simulink model "A12_3_v2018_blagodaram_Ana"  (R2018a)
settings: Solver=ode45  StartTime=0.0  StopTime=300  RelTol=1e-3  EnableMultiTasking=on
libraries: simulink x2
settings Model: Creator=Gorjan  LastModifiedBy=Ana Sofronievska
settings DataIOCC: LimitDataPoints=on  SaveFormat=Array
settings OptimizationCC: LifeSpan=inf
settings DebuggingCC: UnderspecifiedInitializationDetection=Classic  MergeDetectMultiDrivingBlocksExec=none  SolverPrmCheckMsg=warning  StateNameClashWarn=warning  SFUnexpectedBacktrackingDiag=warning  SFNoUnconditionalDefaultTransitionDiag=warning  SFExecutionAtInitializationDiag=none
settings HardwareCC: ProdBitPerPointer=32  ProdBitPerSizeT=32  ProdBitPerPtrDiffT=32  ProdLargestAtomicFloat=None  ProdIntDivRoundTo=Undefined  ProdEndianess=Unspecified  ProdWordSize=32  ProdHWDeviceType=32-bit Generic
settings ModelReferenceCC: PropagateSignalLabelsOutOfModel=off
settings CodeAppCC: StateflowObjectComments=on
settings GRTTargetCC: TargetLangStandard=C89/C90 (ANSI)
settings ConfigComp: CovMetricSettings=dw  CovSaveCumulativeToWorkspaceVar=on  CovSaveSingleToWorkspaceVar=on  CovExternalEMLEnable=off

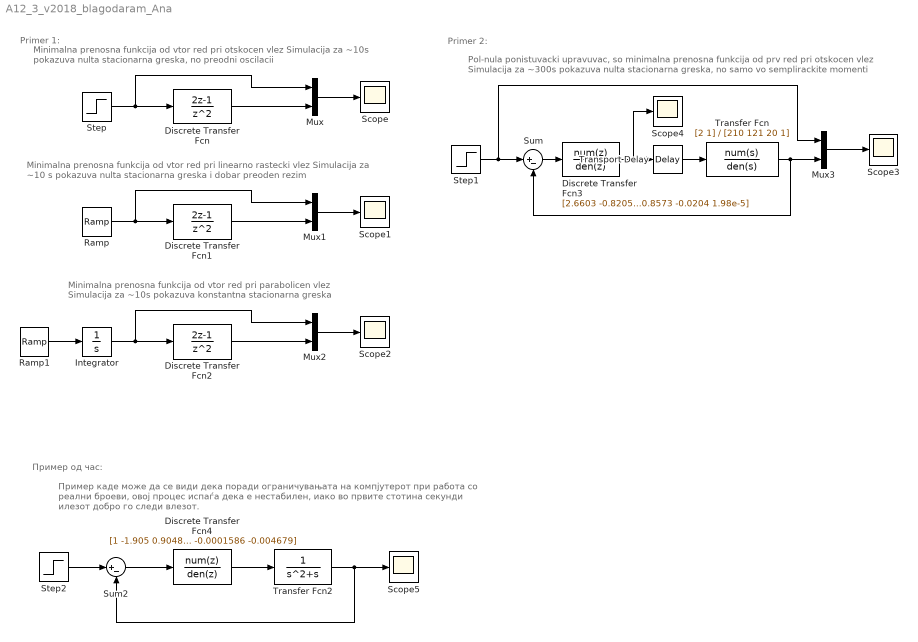
== system A12_3_v2018_blagodaram_Ana ==
  note: Primer 2:
  note: Primer 1:
  note: Minimalna prenosna funkcija od vtor red pri otskocen vlez
      | Simulacija za ~10s pokazuva nulta stacionarna greska, no preodni oscilacii
  note: Minimalna prenosna funkcija od vtor red pri linearno rastecki vlez
      | Simulacija za ~10 s pokazuva nulta stacionarna greska i dobar preoden rezim
  note: Minimalna prenosna funkcija od vtor red pri parabolicen vlez
      | Simulacija za ~10s pokazuva konstantna stacionarna greska
  note: Pol-nula ponistuvacki upravuvac, so minimalna prenosna funkcija od prv red pri otskocen vlez
      | Simulacija za ~300s pokazuva nulta stacionarna greska, no samo vo semplirackite momenti
  note: Пример од час:
  note: Пример каде може да се види дека поради ограничувањата на компјутерот при работа со реални броеви, овој процес испаѓа дека е нестабилен, иако во првите стотина секунди илезот добро го следи влезот.
  Discrete Transfer Fcn : DiscreteTransferFcn  Numerator=[2 -1]  Denominator=[1 0 0]  SampleTime=1
  Discrete Transfer Fcn1 : DiscreteTransferFcn  Numerator=[2 -1]  Denominator=[1 0 0]  SampleTime=1
  Discrete Transfer Fcn2 : DiscreteTransferFcn  Numerator=[2 -1]  Denominator=[1 0 0]  SampleTime=1
  Discrete Transfer Fcn3 : DiscreteTransferFcn  Numerator=[2.6603 -0.8205 0.0585 -2.64e-4 0]  Denominator=[1 -0.1223 -0.8573 -0.0204 1.98e-5]  SampleTime=16
  Discrete Transfer Fcn4 : DiscreteTransferFcn  Numerator=[1 -1.905 0.9048]  Denominator=[0.004837 -0.0001586 -0.004679]  SampleTime=0.1
  Integrator : Integrator
  Mux{,1..3} (4 alike) : Mux  Inputs=2
  Ramp : simulink/Sources/Ramp  slope=1  start=0  InitialOutput=0
  Ramp1 : simulink/Sources/Ramp  slope=1  start=0  InitialOutput=0
  Scope{,1..5} (6 alike) : Scope
  Step : Step  Time=0  SampleTime=0
  Step1 : Step  Time=0  SampleTime=16
  Step2 : Step  SampleTime=0.1
  Sum : Sum  Inputs=|+-  SampleTime=16
  Sum2 : Sum  Inputs=|+-  SampleTime=0.1
  Transfer Fcn : TransferFcn  Numerator=[2 1]  Denominator=[210 121 20 1]
  Transfer Fcn2 : TransferFcn  Denominator=[1 1 0]
  Transport Delay : TransportDelay  DelayTime=4
  wires:
  Step/1 -> Mux/1, Discrete Transfer Fcn/1
  Mux/1 -> Scope/1
  Discrete Transfer Fcn/1 -> Mux/2
  Ramp/1 -> Mux1/1, Discrete Transfer Fcn1/1
  Mux1/1 -> Scope1/1
  Discrete Transfer Fcn1/1 -> Mux1/2
  Ramp1/1 -> Integrator/1
  Mux2/1 -> Scope2/1
  Discrete Transfer Fcn2/1 -> Mux2/2
  Integrator/1 -> Mux2/1, Discrete Transfer Fcn2/1
  Step1/1 -> Mux3/1, Sum/1
  Sum/1 -> Discrete Transfer Fcn3/1
  Discrete Transfer Fcn3/1 -> Scope4/1, Transport Delay/1
  Transfer Fcn/1 -> Sum/2, Mux3/2
  Mux3/1 -> Scope3/1
  Transport Delay/1 -> Transfer Fcn/1
  Step2/1 -> Sum2/1
  Sum2/1 -> Discrete Transfer Fcn4/1
  Discrete Transfer Fcn4/1 -> Transfer Fcn2/1
  Transfer Fcn2/1 -> Sum2/2, Scope5/1
